simulink library "inp"  (Simulink 7.4)
settings: Solver=ode45  StartTime=0.0  StopTime=10.0  RelTol=1e-3
undefined symbols (not defined in the file): AINP_BrkPedalInterp_X_bar, C_TASK_10MS_S, ENUM_SHIFTER_D, ENUM_SHIFTER_N, ENUM_SHIFTER_P, ENUM_SHIFTER_R, KINP_BonnetCloseVehSpdThre_kph, KINP_EDUCoolantTempFilTm_s, KINP_EDUOilPressureFilTm_s, KINP_EDUOilTempFilTm_s, KINP_EDUSynchDisp_mm, KINP_EDUSynchPosnPWMDC_pct_LowerLimit, KINP_EDUSynchPosnPWMDC_pct_ovrdflg, KINP_EDUSynchPosnPWMDC_pct_ovrdval, KINP_EDUSynchPosnPWMDC_pct_UpperLimit, KINP_ShifterPosConfirmD_s, KINP_ShifterPosConfirmN_s, KINP_ShifterPosConfirmP_s, KINP_ShifterPosConfirmR_s, KINP_SingleAccPedalFltRateLim_pct, KINP_TMSpd2VehSpdSigNeg_rpm, KINP_TMSpd2VehSpdSigPos_rpm, KINP_ValidCheck_EDUSynchPosnPWMDC_dec, KINP_ValidCheck_EDUSynchPosnPWMDC_inc, KINP_ValidCheck_EDUSynchPosnPWMDC_lim, KINP_VehSpdSigKeepThres_kph, KPH2MPS, MIN2SEC, MINP_BrkPedalInterp_pct, MPS2KPH, PI, seat_version_control_block_callbacks, TIRE_RADIUS
libraries: inp_lib x166, hcu_lib x4, simulink x1
(part 4 of 9)

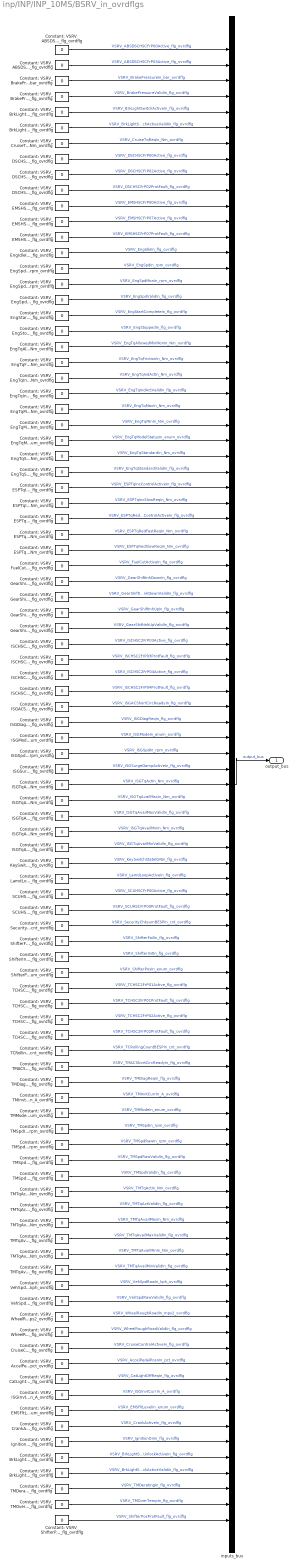
== system inp/INP/INP_10MS/BSRV_in_ovrdflgs ==
  Constant: VSRV_ABSDSCHSCFrP00Active_flg_ovrdflg : Constant  Value=0  OutDataTypeMode=boolean  OutDataTypeStr=boolean
  Constant: VSRV_ABSDSCHSCFrP03Active_flg_ovrdflg : Constant  Value=0  OutDataTypeMode=boolean  OutDataTypeStr=boolean
  Constant: VSRV_AccelPedalPosnIn_pct_ovrdflg : Constant  Value=0  OutDataTypeMode=boolean  OutDataTypeStr=boolean
  Constant: VSRV_BrakePressureIn_bar_ovrdflg : Constant  Value=0  OutDataTypeMode=boolean  OutDataTypeStr=boolean
  Constant: VSRV_BrakePressureValidIn_flg_ovrdflg : Constant  Value=0  OutDataTypeMode=boolean  OutDataTypeStr=boolean
  Constant: VSRV_BrkLightSWPUnlockActiveIn_flg_ovrdflg : Constant  Value=0  OutDataTypeMode=boolean  OutDataTypeStr=boolean
  Constant: VSRV_BrkLightSWPUnlockActiveValidIn_flg_ovrdflg : Constant  Value=0  OutDataTypeMode=boolean  OutDataTypeStr=boolean
  Constant: VSRV_BrkLightSwitchActiveIn_flg_ovrdflg : Constant  Value=0  OutDataTypeMode=boolean  OutDataTypeStr=boolean
  Constant: VSRV_BrkLightSwitchActiveValidIn_flg_ovrdflg : Constant  Value=0  OutDataTypeMode=boolean  OutDataTypeStr=boolean
  Constant: VSRV_CatLightOffReqIn_flg_ovrdflg : Constant  Value=0  OutDataTypeMode=boolean  OutDataTypeStr=boolean
  Constant: VSRV_CrankActiveIn_flg_ovrdflg : Constant  Value=0  OutDataTypeMode=boolean  OutDataTypeStr=boolean
  Constant: VSRV_CruiseControlActiveIn_flg_ovrdflg : Constant  Value=0  OutDataTypeMode=boolean  OutDataTypeStr=boolean
  Constant: VSRV_CruiseTqReqIn_Nm_ovrdflg : Constant  Value=0  OutDataTypeMode=boolean  OutDataTypeStr=boolean
  Constant: VSRV_DSCHSCFrP00Active_flg_ovrdflg : Constant  Value=0  OutDataTypeMode=boolean  OutDataTypeStr=boolean
  Constant: VSRV_DSCHSCFrP02Active_flg_ovrdflg : Constant  Value=0  OutDataTypeMode=boolean  OutDataTypeStr=boolean
  Constant: VSRV_DSCHSCFrP02ProtFault_flg_ovrdflg : Constant  Value=0  OutDataTypeMode=boolean  OutDataTypeStr=boolean
  Constant: VSRV_EMSFltLevelIn_enum_ovrdflg : Constant  Value=0  OutDataTypeMode=boolean  OutDataTypeStr=boolean
  Constant: VSRV_EMSHSCFrP00Active_flg_ovrdflg : Constant  Value=0  OutDataTypeMode=boolean  OutDataTypeStr=boolean
  Constant: VSRV_EMSHSCFrP07Active_flg_ovrdflg : Constant  Value=0  OutDataTypeMode=boolean  OutDataTypeStr=boolean
  Constant: VSRV_EMSHSCFrP07ProtFault_flg_ovrdflg : Constant  Value=0  OutDataTypeMode=boolean  OutDataTypeStr=boolean
  Constant: VSRV_ESPTqIncControlActiveIn_flg_ovrdflg : Constant  Value=0  OutDataTypeMode=boolean  OutDataTypeStr=boolean
  Constant: VSRV_ESPTqIncSlowReqIn_Nm_ovrdflg : Constant  Value=0  OutDataTypeMode=boolean  OutDataTypeStr=boolean
  Constant: VSRV_ESPTqRedControlActiveIn_flg_ovrdflg : Constant  Value=0  OutDataTypeMode=boolean  OutDataTypeStr=boolean
  Constant: VSRV_ESPTqRedFastReqIn_Nm_ovrdflg : Constant  Value=0  OutDataTypeMode=boolean  OutDataTypeStr=boolean
  Constant: VSRV_ESPTqRedSlowReqIn_Nm_ovrdflg : Constant  Value=0  OutDataTypeMode=boolean  OutDataTypeStr=boolean
  Constant: VSRV_EngIdleIn_flg_ovrdflg : Constant  Value=0  OutDataTypeMode=boolean  OutDataTypeStr=boolean
  Constant: VSRV_EngSpdIn_rpm_ovrdflg : Constant  Value=0  OutDataTypeMode=boolean  OutDataTypeStr=boolean
  Constant: VSRV_EngSpdMonIn_rpm_ovrdflg : Constant  Value=0  OutDataTypeMode=boolean  OutDataTypeStr=boolean
  Constant: VSRV_EngSpdValidIn_flg_ovrdflg : Constant  Value=0  OutDataTypeMode=boolean  OutDataTypeStr=boolean
  Constant: VSRV_EngStartCompleteIn_flg_ovrdflg : Constant  Value=0  OutDataTypeMode=boolean  OutDataTypeStr=boolean
  Constant: VSRV_EngStoppedIn_flg_ovrdflg : Constant  Value=0  OutDataTypeMode=boolean  OutDataTypeStr=boolean
  Constant: VSRV_EngTqAllowedMinMonIn_Nm_ovrdflg : Constant  Value=0  OutDataTypeMode=boolean  OutDataTypeStr=boolean
  Constant: VSRV_EngTqFrictionIn_Nm_ovrdflg : Constant  Value=0  OutDataTypeMode=boolean  OutDataTypeStr=boolean
  Constant: VSRV_EngTqIndActIn_Nm_ovrdflg : Constant  Value=0  OutDataTypeMode=boolean  OutDataTypeStr=boolean
  Constant: VSRV_EngTqIndActValidIn_flg_ovrdflg : Constant  Value=0  OutDataTypeMode=boolean  OutDataTypeStr=boolean
  Constant: VSRV_EngTqMaxIn_Nm_ovrdflg : Constant  Value=0  OutDataTypeMode=boolean  OutDataTypeStr=boolean
  Constant: VSRV_EngTqMinIn_Nm_ovrdflg : Constant  Value=0  OutDataTypeMode=boolean  OutDataTypeStr=boolean
  Constant: VSRV_EngTqModelStatusIn_enum_ovrdflg : Constant  Value=0  OutDataTypeMode=boolean  OutDataTypeStr=boolean
  Constant: VSRV_EngTqStandardIn_Nm_ovrdflg : Constant  Value=0  OutDataTypeMode=boolean  OutDataTypeStr=boolean
  Constant: VSRV_EngTqStandardValidIn_flg_ovrdflg : Constant  Value=0  OutDataTypeMode=boolean  OutDataTypeStr=boolean
  Constant: VSRV_FuelCutActiveIn_flg_ovrdflg : Constant  Value=0  OutDataTypeMode=boolean  OutDataTypeStr=boolean
  Constant: VSRV_GearShiftInhDownIn_flg_ovrdflg : Constant  Value=0  OutDataTypeMode=boolean  OutDataTypeStr=boolean
  Constant: VSRV_GearShiftInhDownValidIn_flg_ovrdflg : Constant  Value=0  OutDataTypeMode=boolean  OutDataTypeStr=boolean
  Constant: VSRV_GearShiftInhUpIn_flg_ovrdflg : Constant  Value=0  OutDataTypeMode=boolean  OutDataTypeStr=boolean
  Constant: VSRV_GearShiftInhUpValidIn_flg_ovrdflg : Constant  Value=0  OutDataTypeMode=boolean  OutDataTypeStr=boolean
  Constant: VSRV_ISCHSC2FrP03Active_flg_ovrdflg : Constant  Value=0  OutDataTypeMode=boolean  OutDataTypeStr=boolean
  Constant: VSRV_ISCHSC2FrP03ProtFault_flg_ovrdflg : Constant  Value=0  OutDataTypeMode=boolean  OutDataTypeStr=boolean
  Constant: VSRV_ISCHSC2FrP04Active_flg_ovrdflg : Constant  Value=0  OutDataTypeMode=boolean  OutDataTypeStr=boolean
  Constant: VSRV_ISCHSC2FrP04ProtFault_flg_ovrdflg : Constant  Value=0  OutDataTypeMode=boolean  OutDataTypeStr=boolean
  Constant: VSRV_ISGACShortCircReadyIn_flg_ovrdflg : Constant  Value=0  OutDataTypeMode=boolean  OutDataTypeStr=boolean
  Constant: VSRV_ISGDiagReqIn_flg_ovrdflg : Constant  Value=0  OutDataTypeMode=boolean  OutDataTypeStr=boolean
  Constant: VSRV_ISGInvtCurrIn_A_ovrdflg : Constant  Value=0  OutDataTypeMode=boolean  OutDataTypeStr=boolean
  Constant: VSRV_ISGModeIn_enum_ovrdflg : Constant  Value=0  OutDataTypeMode=boolean  OutDataTypeStr=boolean
  Constant: VSRV_ISGSpdIn_rpm_ovrdflg : Constant  Value=0  OutDataTypeMode=boolean  OutDataTypeStr=boolean
  Constant: VSRV_ISGSurgeDampActiveIn_flg_ovrdflg : Constant  Value=0  OutDataTypeMode=boolean  OutDataTypeStr=boolean
  Constant: VSRV_ISGTqActIn_Nm_ovrdflg : Constant  Value=0  OutDataTypeMode=boolean  OutDataTypeStr=boolean
  Constant: VSRV_ISGTqAvailMaxIn_Nm_ovrdflg : Constant  Value=0  OutDataTypeMode=boolean  OutDataTypeStr=boolean
  Constant: VSRV_ISGTqAvailMaxValidIn_flg_ovrdflg : Constant  Value=0  OutDataTypeMode=boolean  OutDataTypeStr=boolean
  Constant: VSRV_ISGTqAvailMinIn_Nm_ovrdflg : Constant  Value=0  OutDataTypeMode=boolean  OutDataTypeStr=boolean
  Constant: VSRV_ISGTqAvailMinValidIn_flg_ovrdflg : Constant  Value=0  OutDataTypeMode=boolean  OutDataTypeStr=boolean
  Constant: VSRV_IgnitionOnIn_flg_ovrdflg : Constant  Value=0  OutDataTypeMode=boolean  OutDataTypeStr=boolean
  Constant: VSRV_KeySwitchStateIGNIn_flg_ovrdflg : Constant  Value=0  OutDataTypeMode=boolean  OutDataTypeStr=boolean
  Constant: VSRV_LamdLoopActiveIn_flg_ovrdflg : Constant  Value=0  OutDataTypeMode=boolean  OutDataTypeStr=boolean
  Constant: VSRV_SCUHSCFrP00Active_flg_ovrdflg : Constant  Value=0  OutDataTypeMode=boolean  OutDataTypeStr=boolean
  Constant: VSRV_SCUHSCFrP00ProtFault_flg_ovrdflg : Constant  Value=0  OutDataTypeMode=boolean  OutDataTypeStr=boolean
  Constant: VSRV_SecurityChksumBESPIn_cnt_ovrdflg : Constant  Value=0  OutDataTypeMode=boolean  OutDataTypeStr=boolean
  Constant: VSRV_ShifterFailIn_flg_ovrdflg : Constant  Value=0  OutDataTypeMode=boolean  OutDataTypeStr=boolean
  Constant: VSRV_ShifterInitIn_flg_ovrdflg : Constant  Value=0  OutDataTypeMode=boolean  OutDataTypeStr=boolean
  Constant: VSRV_ShifterPosIn_enum_ovrdflg : Constant  Value=0  OutDataTypeMode=boolean  OutDataTypeStr=boolean
  Constant: VSRV_ShifterPosProtFault_flg_ovrdflg : Constant  Value=0  OutDataTypeMode=boolean  OutDataTypeStr=boolean
  Constant: VSRV_TCHSC2FrP01Active_flg_ovrdflg : Constant  Value=0  OutDataTypeMode=boolean  OutDataTypeStr=boolean
  Constant: VSRV_TCHSC2FrP01ProtFault_flg_ovrdflg : Constant  Value=0  OutDataTypeMode=boolean  OutDataTypeStr=boolean
  Constant: VSRV_TCHSC2FrP02Active_flg_ovrdflg : Constant  Value=0  OutDataTypeMode=boolean  OutDataTypeStr=boolean
  Constant: VSRV_TCHSC2FrP02ProtFault_flg_ovrdflg : Constant  Value=0  OutDataTypeMode=boolean  OutDataTypeStr=boolean
  Constant: VSRV_TCRollingCountBESPIn_cnt_ovrdflg : Constant  Value=0  OutDataTypeMode=boolean  OutDataTypeStr=boolean
  Constant: VSRV_TMACShortCircReadyIn_flg_ovrdflg : Constant  Value=0  OutDataTypeMode=boolean  OutDataTypeStr=boolean
  Constant: VSRV_TMDeratingIn_flg_ovrdflg : Constant  Value=0  OutDataTypeMode=boolean  OutDataTypeStr=boolean
  Constant: VSRV_TMDiagReqIn_flg_ovrdflg : Constant  Value=0  OutDataTypeMode=boolean  OutDataTypeStr=boolean
  Constant: VSRV_TMInvtCurrIn_A_ovrdflg : Constant  Value=0  OutDataTypeMode=boolean  OutDataTypeStr=boolean
  Constant: VSRV_TMModeIn_enum_ovrdflg : Constant  Value=0  OutDataTypeMode=boolean  OutDataTypeStr=boolean
  Constant: VSRV_TMOverTempIn_flg_ovrdflg : Constant  Value=0  OutDataTypeMode=boolean  OutDataTypeStr=boolean
  Constant: VSRV_TMSpdIn_rpm_ovrdflg : Constant  Value=0  OutDataTypeMode=boolean  OutDataTypeStr=boolean
  Constant: VSRV_TMSpdRawIn_rpm_ovrdflg : Constant  Value=0  OutDataTypeMode=boolean  OutDataTypeStr=boolean
  Constant: VSRV_TMSpdRawValidIn_flg_ovrdflg : Constant  Value=0  OutDataTypeMode=boolean  OutDataTypeStr=boolean
  Constant: VSRV_TMSpdValidIn_flg_ovrdflg : Constant  Value=0  OutDataTypeMode=boolean  OutDataTypeStr=boolean
  Constant: VSRV_TMTqActIn_Nm_ovrdflg : Constant  Value=0  OutDataTypeMode=boolean  OutDataTypeStr=boolean
  Constant: VSRV_TMTqActValidIn_flg_ovrdflg : Constant  Value=0  OutDataTypeMode=boolean  OutDataTypeStr=boolean
  Constant: VSRV_TMTqAvailMaxIn_Nm_ovrdflg : Constant  Value=0  OutDataTypeMode=boolean  OutDataTypeStr=boolean
  Constant: VSRV_TMTqAvailMaxValidIn_flg_ovrdflg : Constant  Value=0  OutDataTypeMode=boolean  OutDataTypeStr=boolean
  Constant: VSRV_TMTqAvailMinIn_Nm_ovrdflg : Constant  Value=0  OutDataTypeMode=boolean  OutDataTypeStr=boolean
  Constant: VSRV_TMTqAvailMinValidIn_flg_ovrdflg : Constant  Value=0  OutDataTypeMode=boolean  OutDataTypeStr=boolean
  Constant: VSRV_VehSpdRawIn_kph_ovrdflg : Constant  Value=0  OutDataTypeMode=boolean  OutDataTypeStr=boolean
  Constant: VSRV_VehSpdRawValidIn_flg_ovrdflg : Constant  Value=0  OutDataTypeMode=boolean  OutDataTypeStr=boolean
  Constant: VSRV_WheelRoughRoadIn_mps2_ovrdflg : Constant  Value=0  OutDataTypeMode=boolean  OutDataTypeStr=boolean
  Constant: VSRV_WheelRoughRoadValidIn_flg_ovrdflg : Constant  Value=0  OutDataTypeMode=boolean  OutDataTypeStr=boolean
  inputs_bus : BusCreator  Inputs=95
  output_bus : Outport
  wires:
  Constant: VSRV_ShifterPosProtFault_flg_ovrdflg/1 -> inputs_bus/95  "VSRV_ShifterPosProtFault_flg_ovrdflg"
  Constant: VSRV_TMOverTempIn_flg_ovrdflg/1 -> inputs_bus/94  "VSRV_TMOverTempIn_flg_ovrdflg"
  Constant: VSRV_TMDeratingIn_flg_ovrdflg/1 -> inputs_bus/93  "VSRV_TMDeratingIn_flg_ovrdflg"
  Constant: VSRV_BrkLightSWPUnlockActiveValidIn_flg_ovrdflg/1 -> inputs_bus/92  "VSRV_BrkLightSWPUnlockActiveValidIn_flg_ovrdflg"
  Constant: VSRV_BrkLightSWPUnlockActiveIn_flg_ovrdflg/1 -> inputs_bus/91  "VSRV_BrkLightSWPUnlockActiveIn_flg_ovrdflg"
  Constant: VSRV_IgnitionOnIn_flg_ovrdflg/1 -> inputs_bus/90  "VSRV_IgnitionOnIn_flg_ovrdflg"
  Constant: VSRV_CrankActiveIn_flg_ovrdflg/1 -> inputs_bus/89  "VSRV_CrankActiveIn_flg_ovrdflg"
  Constant: VSRV_WheelRoughRoadValidIn_flg_ovrdflg/1 -> inputs_bus/83  "VSRV_WheelRoughRoadValidIn_flg_ovrdflg"
  Constant: VSRV_WheelRoughRoadIn_mps2_ovrdflg/1 -> inputs_bus/82  "VSRV_WheelRoughRoadIn_mps2_ovrdflg"
  Constant: VSRV_VehSpdRawValidIn_flg_ovrdflg/1 -> inputs_bus/81  "VSRV_VehSpdRawValidIn_flg_ovrdflg"
  Constant: VSRV_VehSpdRawIn_kph_ovrdflg/1 -> inputs_bus/80  "VSRV_VehSpdRawIn_kph_ovrdflg"
  Constant: VSRV_TMTqAvailMinValidIn_flg_ovrdflg/1 -> inputs_bus/79  "VSRV_TMTqAvailMinValidIn_flg_ovrdflg"
  Constant: VSRV_TMTqAvailMinIn_Nm_ovrdflg/1 -> inputs_bus/78  "VSRV_TMTqAvailMinIn_Nm_ovrdflg"
  Constant: VSRV_TMTqAvailMaxValidIn_flg_ovrdflg/1 -> inputs_bus/77  "VSRV_TMTqAvailMaxValidIn_flg_ovrdflg"
  Constant: VSRV_TMTqAvailMaxIn_Nm_ovrdflg/1 -> inputs_bus/76  "VSRV_TMTqAvailMaxIn_Nm_ovrdflg"
  Constant: VSRV_TMTqActValidIn_flg_ovrdflg/1 -> inputs_bus/75  "VSRV_TMTqActValidIn_flg_ovrdflg"
  Constant: VSRV_TMTqActIn_Nm_ovrdflg/1 -> inputs_bus/74  "VSRV_TMTqActIn_Nm_ovrdflg"
  Constant: VSRV_TMSpdValidIn_flg_ovrdflg/1 -> inputs_bus/73  "VSRV_TMSpdValidIn_flg_ovrdflg"
  Constant: VSRV_TMSpdRawValidIn_flg_ovrdflg/1 -> inputs_bus/72  "VSRV_TMSpdRawValidIn_flg_ovrdflg"
  Constant: VSRV_TMSpdRawIn_rpm_ovrdflg/1 -> inputs_bus/71  "VSRV_TMSpdRawIn_rpm_ovrdflg"
  Constant: VSRV_TMSpdIn_rpm_ovrdflg/1 -> inputs_bus/70  "VSRV_TMSpdIn_rpm_ovrdflg"
  Constant: VSRV_TMModeIn_enum_ovrdflg/1 -> inputs_bus/69  "VSRV_TMModeIn_enum_ovrdflg"
  Constant: VSRV_TMInvtCurrIn_A_ovrdflg/1 -> inputs_bus/68  "VSRV_TMInvtCurrIn_A_ovrdflg"
  Constant: VSRV_TMDiagReqIn_flg_ovrdflg/1 -> inputs_bus/67  "VSRV_TMDiagReqIn_flg_ovrdflg"
  Constant: VSRV_TMACShortCircReadyIn_flg_ovrdflg/1 -> inputs_bus/66  "VSRV_TMACShortCircReadyIn_flg_ovrdflg"
  Constant: VSRV_TCRollingCountBESPIn_cnt_ovrdflg/1 -> inputs_bus/65  "VSRV_TCRollingCountBESPIn_cnt_ovrdflg"
  Constant: VSRV_TCHSC2FrP02ProtFault_flg_ovrdflg/1 -> inputs_bus/64  "VSRV_TCHSC2FrP02ProtFault_flg_ovrdflg"
  Constant: VSRV_TCHSC2FrP02Active_flg_ovrdflg/1 -> inputs_bus/63  "VSRV_TCHSC2FrP02Active_flg_ovrdflg"
  Constant: VSRV_TCHSC2FrP01ProtFault_flg_ovrdflg/1 -> inputs_bus/62  "VSRV_TCHSC2FrP01ProtFault_flg_ovrdflg"
  Constant: VSRV_TCHSC2FrP01Active_flg_ovrdflg/1 -> inputs_bus/61  "VSRV_TCHSC2FrP01Active_flg_ovrdflg"
  Constant: VSRV_ShifterPosIn_enum_ovrdflg/1 -> inputs_bus/60  "VSRV_ShifterPosIn_enum_ovrdflg"
  Constant: VSRV_ShifterInitIn_flg_ovrdflg/1 -> inputs_bus/59  "VSRV_ShifterInitIn_flg_ovrdflg"
  Constant: VSRV_ShifterFailIn_flg_ovrdflg/1 -> inputs_bus/58  "VSRV_ShifterFailIn_flg_ovrdflg"
  Constant: VSRV_SecurityChksumBESPIn_cnt_ovrdflg/1 -> inputs_bus/57  "VSRV_SecurityChksumBESPIn_cnt_ovrdflg"
  Constant: VSRV_SCUHSCFrP00ProtFault_flg_ovrdflg/1 -> inputs_bus/56  "VSRV_SCUHSCFrP00ProtFault_flg_ovrdflg"
  Constant: VSRV_SCUHSCFrP00Active_flg_ovrdflg/1 -> inputs_bus/55  "VSRV_SCUHSCFrP00Active_flg_ovrdflg"
  Constant: VSRV_LamdLoopActiveIn_flg_ovrdflg/1 -> inputs_bus/54  "VSRV_LamdLoopActiveIn_flg_ovrdflg"
  Constant: VSRV_KeySwitchStateIGNIn_flg_ovrdflg/1 -> inputs_bus/53  "VSRV_KeySwitchStateIGNIn_flg_ovrdflg"
  Constant: VSRV_ISGTqAvailMinValidIn_flg_ovrdflg/1 -> inputs_bus/52  "VSRV_ISGTqAvailMinValidIn_flg_ovrdflg"
  Constant: VSRV_ISGTqAvailMinIn_Nm_ovrdflg/1 -> inputs_bus/51  "VSRV_ISGTqAvailMinIn_Nm_ovrdflg"
  Constant: VSRV_ISGTqAvailMaxValidIn_flg_ovrdflg/1 -> inputs_bus/50  "VSRV_ISGTqAvailMaxValidIn_flg_ovrdflg"
  Constant: VSRV_ISGTqAvailMaxIn_Nm_ovrdflg/1 -> inputs_bus/49  "VSRV_ISGTqAvailMaxIn_Nm_ovrdflg"
  Constant: VSRV_ISGTqActIn_Nm_ovrdflg/1 -> inputs_bus/48  "VSRV_ISGTqActIn_Nm_ovrdflg"
  Constant: VSRV_ISGSurgeDampActiveIn_flg_ovrdflg/1 -> inputs_bus/47  "VSRV_ISGSurgeDampActiveIn_flg_ovrdflg"
  Constant: VSRV_ISGSpdIn_rpm_ovrdflg/1 -> inputs_bus/46  "VSRV_ISGSpdIn_rpm_ovrdflg"
  Constant: VSRV_ISGModeIn_enum_ovrdflg/1 -> inputs_bus/45  "VSRV_ISGModeIn_enum_ovrdflg"
  Constant: VSRV_ISGDiagReqIn_flg_ovrdflg/1 -> inputs_bus/44  "VSRV_ISGDiagReqIn_flg_ovrdflg"
  Constant: VSRV_ISGACShortCircReadyIn_flg_ovrdflg/1 -> inputs_bus/43  "VSRV_ISGACShortCircReadyIn_flg_ovrdflg"
  Constant: VSRV_ISCHSC2FrP04ProtFault_flg_ovrdflg/1 -> inputs_bus/42  "VSRV_ISCHSC2FrP04ProtFault_flg_ovrdflg"
  Constant: VSRV_ISCHSC2FrP04Active_flg_ovrdflg/1 -> inputs_bus/41  "VSRV_ISCHSC2FrP04Active_flg_ovrdflg"
  Constant: VSRV_ISCHSC2FrP03ProtFault_flg_ovrdflg/1 -> inputs_bus/40  "VSRV_ISCHSC2FrP03ProtFault_flg_ovrdflg"
  Constant: VSRV_ISCHSC2FrP03Active_flg_ovrdflg/1 -> inputs_bus/39  "VSRV_ISCHSC2FrP03Active_flg_ovrdflg"
  Constant: VSRV_GearShiftInhUpValidIn_flg_ovrdflg/1 -> inputs_bus/38  "VSRV_GearShiftInhUpValidIn_flg_ovrdflg"
  Constant: VSRV_GearShiftInhUpIn_flg_ovrdflg/1 -> inputs_bus/37  "VSRV_GearShiftInhUpIn_flg_ovrdflg"
  Constant: VSRV_GearShiftInhDownValidIn_flg_ovrdflg/1 -> inputs_bus/36  "VSRV_GearShiftInhDownValidIn_flg_ovrdflg"
  Constant: VSRV_GearShiftInhDownIn_flg_ovrdflg/1 -> inputs_bus/35  "VSRV_GearShiftInhDownIn_flg_ovrdflg"
  Constant: VSRV_FuelCutActiveIn_flg_ovrdflg/1 -> inputs_bus/34  "VSRV_FuelCutActiveIn_flg_ovrdflg"
  Constant: VSRV_ESPTqRedSlowReqIn_Nm_ovrdflg/1 -> inputs_bus/33  "VSRV_ESPTqRedSlowReqIn_Nm_ovrdflg"
  Constant: VSRV_ESPTqRedFastReqIn_Nm_ovrdflg/1 -> inputs_bus/32  "VSRV_ESPTqRedFastReqIn_Nm_ovrdflg"
  Constant: VSRV_ESPTqRedControlActiveIn_flg_ovrdflg/1 -> inputs_bus/31  "VSRV_ESPTqRedControlActiveIn_flg_ovrdflg"
  Constant: VSRV_ESPTqIncSlowReqIn_Nm_ovrdflg/1 -> inputs_bus/30  "VSRV_ESPTqIncSlowReqIn_Nm_ovrdflg"
  Constant: VSRV_ESPTqIncControlActiveIn_flg_ovrdflg/1 -> inputs_bus/29  "VSRV_ESPTqIncControlActiveIn_flg_ovrdflg"
  Constant: VSRV_EngTqStandardValidIn_flg_ovrdflg/1 -> inputs_bus/28  "VSRV_EngTqStandardValidIn_flg_ovrdflg"
  Constant: VSRV_EngTqStandardIn_Nm_ovrdflg/1 -> inputs_bus/27  "VSRV_EngTqStandardIn_Nm_ovrdflg"
  Constant: VSRV_EngTqModelStatusIn_enum_ovrdflg/1 -> inputs_bus/26  "VSRV_EngTqModelStatusIn_enum_ovrdflg"
  Constant: VSRV_EngTqMinIn_Nm_ovrdflg/1 -> inputs_bus/25  "VSRV_EngTqMinIn_Nm_ovrdflg"
  Constant: VSRV_EngTqMaxIn_Nm_ovrdflg/1 -> inputs_bus/24  "VSRV_EngTqMaxIn_Nm_ovrdflg"
  Constant: VSRV_EngTqIndActValidIn_flg_ovrdflg/1 -> inputs_bus/23  "VSRV_EngTqIndActValidIn_flg_ovrdflg"
  Constant: VSRV_EngTqIndActIn_Nm_ovrdflg/1 -> inputs_bus/22  "VSRV_EngTqIndActIn_Nm_ovrdflg"
  Constant: VSRV_EngTqFrictionIn_Nm_ovrdflg/1 -> inputs_bus/21  "VSRV_EngTqFrictionIn_Nm_ovrdflg"
  Constant: VSRV_EngTqAllowedMinMonIn_Nm_ovrdflg/1 -> inputs_bus/20  "VSRV_EngTqAllowedMinMonIn_Nm_ovrdflg"
  Constant: VSRV_EngStoppedIn_flg_ovrdflg/1 -> inputs_bus/19  "VSRV_EngStoppedIn_flg_ovrdflg"
  Constant: VSRV_EngStartCompleteIn_flg_ovrdflg/1 -> inputs_bus/18  "VSRV_EngStartCompleteIn_flg_ovrdflg"
  Constant: VSRV_EngSpdValidIn_flg_ovrdflg/1 -> inputs_bus/17  "VSRV_EngSpdValidIn_flg_ovrdflg"
  Constant: VSRV_EngSpdMonIn_rpm_ovrdflg/1 -> inputs_bus/16  "VSRV_EngSpdMonIn_rpm_ovrdflg"
  Constant: VSRV_EngSpdIn_rpm_ovrdflg/1 -> inputs_bus/15  "VSRV_EngSpdIn_rpm_ovrdflg"
  Constant: VSRV_EngIdleIn_flg_ovrdflg/1 -> inputs_bus/14  "VSRV_EngIdleIn_flg_ovrdflg"
  Constant: VSRV_EMSHSCFrP07ProtFault_flg_ovrdflg/1 -> inputs_bus/13  "VSRV_EMSHSCFrP07ProtFault_flg_ovrdflg"
  Constant: VSRV_EMSHSCFrP07Active_flg_ovrdflg/1 -> inputs_bus/12  "VSRV_EMSHSCFrP07Active_flg_ovrdflg"
  Constant: VSRV_EMSHSCFrP00Active_flg_ovrdflg/1 -> inputs_bus/11  "VSRV_EMSHSCFrP00Active_flg_ovrdflg"
  Constant: VSRV_DSCHSCFrP02ProtFault_flg_ovrdflg/1 -> inputs_bus/10  "VSRV_DSCHSCFrP02ProtFault_flg_ovrdflg"
  Constant: VSRV_DSCHSCFrP02Active_flg_ovrdflg/1 -> inputs_bus/9  "VSRV_DSCHSCFrP02Active_flg_ovrdflg"
  Constant: VSRV_DSCHSCFrP00Active_flg_ovrdflg/1 -> inputs_bus/8  "VSRV_DSCHSCFrP00Active_flg_ovrdflg"
  Constant: VSRV_CruiseTqReqIn_Nm_ovrdflg/1 -> inputs_bus/7  "VSRV_CruiseTqReqIn_Nm_ovrdflg"
  Constant: VSRV_BrkLightSwitchActiveValidIn_flg_ovrdflg/1 -> inputs_bus/6  "VSRV_BrkLightSwitchActiveValidIn_flg_ovrdflg"
  Constant: VSRV_BrkLightSwitchActiveIn_flg_ovrdflg/1 -> inputs_bus/5  "VSRV_BrkLightSwitchActiveIn_flg_ovrdflg"
  Constant: VSRV_BrakePressureValidIn_flg_ovrdflg/1 -> inputs_bus/4  "VSRV_BrakePressureValidIn_flg_ovrdflg"
  Constant: VSRV_BrakePressureIn_bar_ovrdflg/1 -> inputs_bus/3  "VSRV_BrakePressureIn_bar_ovrdflg"
  Constant: VSRV_ABSDSCHSCFrP03Active_flg_ovrdflg/1 -> inputs_bus/2  "VSRV_ABSDSCHSCFrP03Active_flg_ovrdflg"
  Constant: VSRV_ABSDSCHSCFrP00Active_flg_ovrdflg/1 -> inputs_bus/1  "VSRV_ABSDSCHSCFrP00Active_flg_ovrdflg"
  inputs_bus/1 -> output_bus/1  "output_bus"
  Constant: VSRV_CruiseControlActiveIn_flg_ovrdflg/1 -> inputs_bus/84  "VSRV_CruiseControlActiveIn_flg_ovrdflg"
  Constant: VSRV_AccelPedalPosnIn_pct_ovrdflg/1 -> inputs_bus/85  "VSRV_AccelPedalPosnIn_pct_ovrdflg"
  Constant: VSRV_CatLightOffReqIn_flg_ovrdflg/1 -> inputs_bus/86  "VSRV_CatLightOffReqIn_flg_ovrdflg"
  Constant: VSRV_ISGInvtCurrIn_A_ovrdflg/1 -> inputs_bus/87  "VSRV_ISGInvtCurrIn_A_ovrdflg"
  Constant: VSRV_EMSFltLevelIn_enum_ovrdflg/1 -> inputs_bus/88  "VSRV_EMSFltLevelIn_enum_ovrdflg"

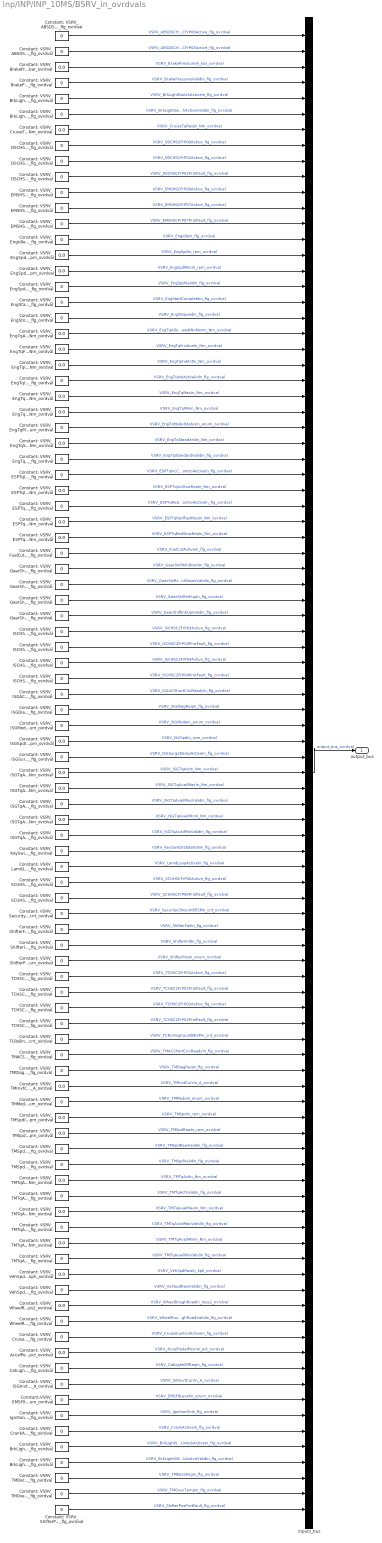
== system inp/INP/INP_10MS/BSRV_in_ovrdvals ==
  Constant: VSRV_ABSDSCHSCFrP00Active_flg_ovrdval : Constant  Value=0  OutDataTypeMode=boolean  OutDataTypeStr=boolean
  Constant: VSRV_ABSDSCHSCFrP03Active_flg_ovrdval : Constant  Value=0  OutDataTypeMode=boolean  OutDataTypeStr=boolean
  Constant: VSRV_AccelPedalPosnMonIn_pct_ovrdval : Constant  Value=0.0  OutDataTypeMode=single  OutDataTypeStr=single
  Constant: VSRV_BrakePressureIn_bar_ovrdval : Constant  Value=0.0  OutDataTypeMode=single  OutDataTypeStr=single
  Constant: VSRV_BrakePressureValidIn_flg_ovrdval : Constant  Value=0  OutDataTypeMode=boolean  OutDataTypeStr=boolean
  Constant: VSRV_BrkLightSWPUnlockActiveIn_flg_ovrdval : Constant  Value=0  OutDataTypeMode=boolean  OutDataTypeStr=boolean
  Constant: VSRV_BrkLightSWPUnlockActiveValidIn_flg_ovrdval : Constant  Value=0  OutDataTypeMode=boolean  OutDataTypeStr=boolean
  Constant: VSRV_BrkLightSwitchActiveIn_flg_ovrdval : Constant  Value=0  OutDataTypeMode=boolean  OutDataTypeStr=boolean
  Constant: VSRV_BrkLightSwitchActiveValidIn_flg_ovrdval : Constant  Value=0  OutDataTypeMode=boolean  OutDataTypeStr=boolean
  Constant: VSRV_CatLightOffReqIn_flg_ovrdval : Constant  Value=0  OutDataTypeMode=boolean  OutDataTypeStr=boolean
  Constant: VSRV_CrankActiveIn_flg_ovrdval : Constant  Value=0  OutDataTypeMode=boolean  OutDataTypeStr=boolean
  Constant: VSRV_CruiseControlActiveIn_flg_ovrdval : Constant  Value=0  OutDataTypeMode=boolean  OutDataTypeStr=boolean
  Constant: VSRV_CruiseTqReqIn_Nm_ovrdval : Constant  Value=0.0  OutDataTypeMode=single  OutDataTypeStr=single
  Constant: VSRV_DSCHSCFrP00Active_flg_ovrdval : Constant  Value=0  OutDataTypeMode=boolean  OutDataTypeStr=boolean
  Constant: VSRV_DSCHSCFrP02Active_flg_ovrdval : Constant  Value=0  OutDataTypeMode=boolean  OutDataTypeStr=boolean
  Constant: VSRV_DSCHSCFrP02ProtFault_flg_ovrdval : Constant  Value=0  OutDataTypeMode=boolean  OutDataTypeStr=boolean
  Constant: VSRV_EMSHSCFrP00Active_flg_ovrdval : Constant  Value=0  OutDataTypeMode=boolean  OutDataTypeStr=boolean
  Constant: VSRV_EMSHSCFrP07Active_flg_ovrdval : Constant  Value=0  OutDataTypeMode=boolean  OutDataTypeStr=boolean
  Constant: VSRV_EMSHSCFrP07ProtFault_flg_ovrdval : Constant  Value=0  OutDataTypeMode=boolean  OutDataTypeStr=boolean
  Constant: VSRV_ESPTqIncControlActiveIn_flg_ovrdval : Constant  Value=0  OutDataTypeMode=boolean  OutDataTypeStr=boolean
  Constant: VSRV_ESPTqIncSlowReqIn_Nm_ovrdval : Constant  Value=0.0  OutDataTypeMode=single  OutDataTypeStr=single
  Constant: VSRV_ESPTqRedControlActiveIn_flg_ovrdval : Constant  Value=0  OutDataTypeMode=boolean  OutDataTypeStr=boolean
  Constant: VSRV_ESPTqRedFastReqIn_Nm_ovrdval : Constant  Value=0.0  OutDataTypeMode=single  OutDataTypeStr=single
  Constant: VSRV_ESPTqRedSlowReqIn_Nm_ovrdval : Constant  Value=0.0  OutDataTypeMode=single  OutDataTypeStr=single
  Constant: VSRV_EngIdleIn_flg_ovrdval : Constant  Value=0  OutDataTypeMode=boolean  OutDataTypeStr=boolean
  Constant: VSRV_EngSpdIn_rpm_ovrdval : Constant  Value=0.0  OutDataTypeMode=single  OutDataTypeStr=single
  Constant: VSRV_EngSpdMonIn_rpm_ovrdval : Constant  Value=0.0  OutDataTypeMode=single  OutDataTypeStr=single
  Constant: VSRV_EngSpdValidIn_flg_ovrdval : Constant  Value=0  OutDataTypeMode=boolean  OutDataTypeStr=boolean
  Constant: VSRV_EngStartCompleteIn_flg_ovrdval : Constant  Value=0  OutDataTypeMode=boolean  OutDataTypeStr=boolean
  Constant: VSRV_EngStoppedIn_flg_ovrdval : Constant  Value=0  OutDataTypeMode=boolean  OutDataTypeStr=boolean
  Constant: VSRV_EngTqAllowedMinMonIn_Nm_ovrdval : Constant  Value=0.0  OutDataTypeMode=single  OutDataTypeStr=single
  Constant: VSRV_EngTqFrictionIn_Nm_ovrdval : Constant  Value=0.0  OutDataTypeMode=single  OutDataTypeStr=single
  Constant: VSRV_EngTqIndActIn_Nm_ovrdval : Constant  Value=0.0  OutDataTypeMode=single  OutDataTypeStr=single
  Constant: VSRV_EngTqIndActValidIn_flg_ovrdval : Constant  Value=0  OutDataTypeMode=boolean  OutDataTypeStr=boolean
  Constant: VSRV_EngTqMaxIn_Nm_ovrdval : Constant  Value=0.0  OutDataTypeMode=single  OutDataTypeStr=single
  Constant: VSRV_EngTqMinIn_Nm_ovrdval : Constant  Value=0.0  OutDataTypeMode=single  OutDataTypeStr=single
  Constant: VSRV_EngTqModelStatusIn_enum_ovrdval : Constant  Value=0  OutDataTypeMode=uint8  OutDataTypeStr=uint8
  Constant: VSRV_EngTqStandardIn_Nm_ovrdval : Constant  Value=0.0  OutDataTypeMode=single  OutDataTypeStr=single
  Constant: VSRV_EngTqStandardValidIn_flg_ovrdval : Constant  Value=0  OutDataTypeMode=boolean  OutDataTypeStr=boolean
  Constant: VSRV_FuelCutActiveIn_flg_ovrdval : Constant  Value=0  OutDataTypeMode=boolean  OutDataTypeStr=boolean
  Constant: VSRV_GearShiftInhDownIn_flg_ovrdval : Constant  Value=0  OutDataTypeMode=boolean  OutDataTypeStr=boolean
  Constant: VSRV_GearShiftInhDownValidIn_flg_ovrdval : Constant  Value=0  OutDataTypeMode=boolean  OutDataTypeStr=boolean
  Constant: VSRV_GearShiftInhUpIn_flg_ovrdval : Constant  Value=0  OutDataTypeMode=boolean  OutDataTypeStr=boolean
  Constant: VSRV_GearShiftInhUpValidIn_flg_ovrdval : Constant  Value=0  OutDataTypeMode=boolean  OutDataTypeStr=boolean
  Constant: VSRV_ISCHSC2FrP03Active_flg_ovrdval : Constant  Value=0  OutDataTypeMode=boolean  OutDataTypeStr=boolean
  Constant: VSRV_ISCHSC2FrP03ProtFault_flg_ovrdval : Constant  Value=0  OutDataTypeMode=boolean  OutDataTypeStr=boolean
  Constant: VSRV_ISCHSC2FrP04Active_flg_ovrdval : Constant  Value=0  OutDataTypeMode=boolean  OutDataTypeStr=boolean
  Constant: VSRV_ISCHSC2FrP04ProtFault_flg_ovrdval : Constant  Value=0  OutDataTypeMode=boolean  OutDataTypeStr=boolean
  Constant: VSRV_ISGACShortCircReadyIn_flg_ovrdval : Constant  Value=0  OutDataTypeMode=boolean  OutDataTypeStr=boolean
  Constant: VSRV_ISGDiagReqIn_flg_ovrdval : Constant  Value=0  OutDataTypeMode=boolean  OutDataTypeStr=boolean
  Constant: VSRV_ISGInvtCurrIn_A_ovrdval : Constant  Value=0  OutDataTypeMode=single  OutDataTypeStr=single
  Constant: VSRV_ISGModeIn_enum_ovrdval : Constant  Value=0  OutDataTypeMode=uint8  OutDataTypeStr=uint8
  Constant: VSRV_ISGSpdIn_rpm_ovrdval : Constant  Value=0.0  OutDataTypeMode=single  OutDataTypeStr=single
  Constant: VSRV_ISGSurgeDampActiveIn_flg_ovrdval : Constant  Value=0  OutDataTypeMode=boolean  OutDataTypeStr=boolean
  Constant: VSRV_ISGTqActIn_Nm_ovrdval : Constant  Value=0.0  OutDataTypeMode=single  OutDataTypeStr=single
  Constant: VSRV_ISGTqAvailMaxIn_Nm_ovrdval : Constant  Value=0.0  OutDataTypeMode=single  OutDataTypeStr=single
  Constant: VSRV_ISGTqAvailMaxValidIn_flg_ovrdval : Constant  Value=0  OutDataTypeMode=boolean  OutDataTypeStr=boolean
  Constant: VSRV_ISGTqAvailMinIn_Nm_ovrdval : Constant  Value=0.0  OutDataTypeMode=single  OutDataTypeStr=single
  Constant: VSRV_ISGTqAvailMinValidIn_flg_ovrdval : Constant  Value=0  OutDataTypeMode=boolean  OutDataTypeStr=boolean
  Constant: VSRV_IgnitionOnIn_flg_ovrdval : Constant  Value=0  OutDataTypeMode=boolean  OutDataTypeStr=boolean
  Constant: VSRV_KeySwitchStateIGNIn_flg_ovrdval : Constant  Value=0  OutDataTypeMode=boolean  OutDataTypeStr=boolean
  Constant: VSRV_LamdLoopActiveIn_flg_ovrdval : Constant  Value=0  OutDataTypeMode=boolean  OutDataTypeStr=boolean
  Constant: VSRV_SCUHSCFrP00Active_flg_ovrdval : Constant  Value=0  OutDataTypeMode=boolean  OutDataTypeStr=boolean
  Constant: VSRV_SCUHSCFrP00ProtFault_flg_ovrdval : Constant  Value=0  OutDataTypeMode=boolean  OutDataTypeStr=boolean
  Constant: VSRV_SecurityChksumBESPIn_cnt_ovrdval : Constant  Value=0  OutDataTypeMode=uint8  OutDataTypeStr=uint8
  Constant: VSRV_ShifterFailIn_flg_ovrdval : Constant  Value=0  OutDataTypeMode=boolean  OutDataTypeStr=boolean
  Constant: VSRV_ShifterInitIn_flg_ovrdval : Constant  Value=0  OutDataTypeMode=boolean  OutDataTypeStr=boolean
  Constant: VSRV_ShifterPosIn_enum_ovrdval : Constant  Value=0  OutDataTypeMode=uint8  OutDataTypeStr=uint8
  Constant: VSRV_ShifterPosProtFault_flg_ovrdval : Constant  Value=0  OutDataTypeMode=boolean  OutDataTypeStr=boolean
  Constant: VSRV_TCHSC2FrP01Active_flg_ovrdval : Constant  Value=0  OutDataTypeMode=boolean  OutDataTypeStr=boolean
  Constant: VSRV_TCHSC2FrP01ProtFault_flg_ovrdval : Constant  Value=0  OutDataTypeMode=boolean  OutDataTypeStr=boolean
  Constant: VSRV_TCHSC2FrP02Active_flg_ovrdval : Constant  Value=0  OutDataTypeMode=boolean  OutDataTypeStr=boolean
  Constant: VSRV_TCHSC2FrP02ProtFault_flg_ovrdval : Constant  Value=0  OutDataTypeMode=boolean  OutDataTypeStr=boolean
  Constant: VSRV_TCRollingCountBESPIn_cnt_ovrdval : Constant  Value=0  OutDataTypeMode=uint8  OutDataTypeStr=uint8
  Constant: VSRV_TMACShortCircReadyIn_flg_ovrdval : Constant  Value=0  OutDataTypeMode=boolean  OutDataTypeStr=boolean
  Constant: VSRV_TMDeratingIn_flg_ovrdval : Constant  Value=0  OutDataTypeMode=boolean  OutDataTypeStr=boolean
  Constant: VSRV_TMDiagReqIn_flg_ovrdval : Constant  Value=0  OutDataTypeMode=boolean  OutDataTypeStr=boolean
  Constant: VSRV_TMInvtCurrIn_A_ovrdval : Constant  Value=0.0  OutDataTypeMode=single  OutDataTypeStr=single
  Constant: VSRV_TMModeIn_enum_ovrdval : Constant  Value=0  OutDataTypeMode=uint8  OutDataTypeStr=uint8
  Constant: VSRV_TMOverTempIn_flg_ovrdval : Constant  Value=0  OutDataTypeMode=boolean  OutDataTypeStr=boolean
  Constant: VSRV_TMSpdIn_rpm_ovrdval : Constant  Value=0.0  OutDataTypeMode=single  OutDataTypeStr=single
  Constant: VSRV_TMSpdRawIn_rpm_ovrdval : Constant  Value=0.0  OutDataTypeMode=single  OutDataTypeStr=single
  Constant: VSRV_TMSpdRawValidIn_flg_ovrdval : Constant  Value=0  OutDataTypeMode=boolean  OutDataTypeStr=boolean
  Constant: VSRV_TMSpdValidIn_flg_ovrdval : Constant  Value=0  OutDataTypeMode=boolean  OutDataTypeStr=boolean
  Constant: VSRV_TMTqActIn_Nm_ovrdval : Constant  Value=0.0  OutDataTypeMode=single  OutDataTypeStr=single
  Constant: VSRV_TMTqActValidIn_flg_ovrdval : Constant  Value=0  OutDataTypeMode=boolean  OutDataTypeStr=boolean
  Constant: VSRV_TMTqAvailMaxIn_Nm_ovrdval : Constant  Value=0.0  OutDataTypeMode=single  OutDataTypeStr=single
  Constant: VSRV_TMTqAvailMaxValidIn_flg_ovrdval : Constant  Value=0  OutDataTypeMode=boolean  OutDataTypeStr=boolean
  Constant: VSRV_TMTqAvailMinIn_Nm_ovrdval : Constant  Value=0.0  OutDataTypeMode=single  OutDataTypeStr=single
  Constant: VSRV_TMTqAvailMinValidIn_flg_ovrdval : Constant  Value=0  OutDataTypeMode=boolean  OutDataTypeStr=boolean
  Constant: VSRV_VehSpdRawIn_kph_ovrdval : Constant  Value=0.0  OutDataTypeMode=single  OutDataTypeStr=single
  Constant: VSRV_VehSpdRawValidIn_flg_ovrdval : Constant  Value=0  OutDataTypeMode=boolean  OutDataTypeStr=boolean
  Constant: VSRV_WheelRoughRoadIn_mps2_ovrdval : Constant  Value=0.0  OutDataTypeMode=single  OutDataTypeStr=single
  Constant: VSRV_WheelRoughRoadValidIn_flg_ovrdval : Constant  Value=0  OutDataTypeMode=boolean  OutDataTypeStr=boolean
  Constant:VSRV_EMSFltLevelIn_enum_ovrdval : Constant  Value=0  OutDataTypeMode=uint8  OutDataTypeStr=uint8
  inputs_bus : BusCreator  Inputs=95
  output_bus : Outport
  wires:
  Constant: VSRV_ShifterPosProtFault_flg_ovrdval/1 -> inputs_bus/95  "VSRV_ShifterPosProtFault_flg_ovrdval"
  Constant: VSRV_TMOverTempIn_flg_ovrdval/1 -> inputs_bus/94  "VSRV_TMOverTempIn_flg_ovrdval"
  Constant: VSRV_TMDeratingIn_flg_ovrdval/1 -> inputs_bus/93  "VSRV_TMDeratingIn_flg_ovrdval"
  Constant: VSRV_BrkLightSWPUnlockActiveValidIn_flg_ovrdval/1 -> inputs_bus/92  "VSRV_BrkLightSWPUnlockActiveValidIn_flg_ovrdval"
  Constant: VSRV_BrkLightSWPUnlockActiveIn_flg_ovrdval/1 -> inputs_bus/91  "VSRV_BrkLightSWPUnlockActiveIn_flg_ovrdval"
  Constant: VSRV_WheelRoughRoadValidIn_flg_ovrdval/1 -> inputs_bus/83  "VSRV_WheelRoughRoadValidIn_flg_ovrdval"
  Constant: VSRV_WheelRoughRoadIn_mps2_ovrdval/1 -> inputs_bus/82  "VSRV_WheelRoughRoadIn_mps2_ovrdval"
  Constant: VSRV_VehSpdRawValidIn_flg_ovrdval/1 -> inputs_bus/81  "VSRV_VehSpdRawValidIn_flg_ovrdval"
  Constant: VSRV_VehSpdRawIn_kph_ovrdval/1 -> inputs_bus/80  "VSRV_VehSpdRawIn_kph_ovrdval"
  Constant: VSRV_TMTqAvailMinValidIn_flg_ovrdval/1 -> inputs_bus/79  "VSRV_TMTqAvailMinValidIn_flg_ovrdval"
  Constant: VSRV_TMTqAvailMinIn_Nm_ovrdval/1 -> inputs_bus/78  "VSRV_TMTqAvailMinIn_Nm_ovrdval"
  Constant: VSRV_TMTqAvailMaxValidIn_flg_ovrdval/1 -> inputs_bus/77  "VSRV_TMTqAvailMaxValidIn_flg_ovrdval"
  Constant: VSRV_TMTqAvailMaxIn_Nm_ovrdval/1 -> inputs_bus/76  "VSRV_TMTqAvailMaxIn_Nm_ovrdval"
  Constant: VSRV_TMTqActValidIn_flg_ovrdval/1 -> inputs_bus/75  "VSRV_TMTqActValidIn_flg_ovrdval"
  Constant: VSRV_TMTqActIn_Nm_ovrdval/1 -> inputs_bus/74  "VSRV_TMTqActIn_Nm_ovrdval"
  Constant: VSRV_TMSpdValidIn_flg_ovrdval/1 -> inputs_bus/73  "VSRV_TMSpdValidIn_flg_ovrdval"
  Constant: VSRV_TMSpdRawValidIn_flg_ovrdval/1 -> inputs_bus/72  "VSRV_TMSpdRawValidIn_flg_ovrdval"
  Constant: VSRV_TMSpdRawIn_rpm_ovrdval/1 -> inputs_bus/71  "VSRV_TMSpdRawIn_rpm_ovrdval"
  Constant: VSRV_TMSpdIn_rpm_ovrdval/1 -> inputs_bus/70  "VSRV_TMSpdIn_rpm_ovrdval"
  Constant: VSRV_TMModeIn_enum_ovrdval/1 -> inputs_bus/69  "VSRV_TMModeIn_enum_ovrdval"
  Constant: VSRV_TMInvtCurrIn_A_ovrdval/1 -> inputs_bus/68  "VSRV_TMInvtCurrIn_A_ovrdval"
  Constant: VSRV_TMDiagReqIn_flg_ovrdval/1 -> inputs_bus/67  "VSRV_TMDiagReqIn_flg_ovrdval"
  Constant: VSRV_TMACShortCircReadyIn_flg_ovrdval/1 -> inputs_bus/66  "VSRV_TMACShortCircReadyIn_flg_ovrdval"
  Constant: VSRV_TCRollingCountBESPIn_cnt_ovrdval/1 -> inputs_bus/65  "VSRV_TCRollingCountBESPIn_cnt_ovrdval"
  Constant: VSRV_TCHSC2FrP02ProtFault_flg_ovrdval/1 -> inputs_bus/64  "VSRV_TCHSC2FrP02ProtFault_flg_ovrdval"
  Constant: VSRV_TCHSC2FrP02Active_flg_ovrdval/1 -> inputs_bus/63  "VSRV_TCHSC2FrP02Active_flg_ovrdval"
  Constant: VSRV_TCHSC2FrP01ProtFault_flg_ovrdval/1 -> inputs_bus/62  "VSRV_TCHSC2FrP01ProtFault_flg_ovrdval"
  Constant: VSRV_TCHSC2FrP01Active_flg_ovrdval/1 -> inputs_bus/61  "VSRV_TCHSC2FrP01Active_flg_ovrdval"
  Constant: VSRV_ShifterPosIn_enum_ovrdval/1 -> inputs_bus/60  "VSRV_ShifterPosIn_enum_ovrdval"
  Constant: VSRV_ShifterInitIn_flg_ovrdval/1 -> inputs_bus/59  "VSRV_ShifterInitIn_flg_ovrdval"
  Constant: VSRV_ShifterFailIn_flg_ovrdval/1 -> inputs_bus/58  "VSRV_ShifterFailIn_flg_ovrdval"
  Constant: VSRV_SecurityChksumBESPIn_cnt_ovrdval/1 -> inputs_bus/57  "VSRV_SecurityChksumBESPIn_cnt_ovrdval"
  Constant: VSRV_SCUHSCFrP00ProtFault_flg_ovrdval/1 -> inputs_bus/56  "VSRV_SCUHSCFrP00ProtFault_flg_ovrdval"
  Constant: VSRV_SCUHSCFrP00Active_flg_ovrdval/1 -> inputs_bus/55  "VSRV_SCUHSCFrP00Active_flg_ovrdval"
  Constant: VSRV_LamdLoopActiveIn_flg_ovrdval/1 -> inputs_bus/54  "VSRV_LamdLoopActiveIn_flg_ovrdval"
  Constant: VSRV_KeySwitchStateIGNIn_flg_ovrdval/1 -> inputs_bus/53  "VSRV_KeySwitchStateIGNIn_flg_ovrdval"
  Constant: VSRV_ISGTqAvailMinValidIn_flg_ovrdval/1 -> inputs_bus/52  "VSRV_ISGTqAvailMinValidIn_flg_ovrdval"
  Constant: VSRV_ISGTqAvailMinIn_Nm_ovrdval/1 -> inputs_bus/51  "VSRV_ISGTqAvailMinIn_Nm_ovrdval"
  Constant: VSRV_ISGTqAvailMaxValidIn_flg_ovrdval/1 -> inputs_bus/50  "VSRV_ISGTqAvailMaxValidIn_flg_ovrdval"
  Constant: VSRV_ISGTqAvailMaxIn_Nm_ovrdval/1 -> inputs_bus/49  "VSRV_ISGTqAvailMaxIn_Nm_ovrdval"
  Constant: VSRV_ISGTqActIn_Nm_ovrdval/1 -> inputs_bus/48  "VSRV_ISGTqActIn_Nm_ovrdval"
  Constant: VSRV_ISGSurgeDampActiveIn_flg_ovrdval/1 -> inputs_bus/47  "VSRV_ISGSurgeDampActiveIn_flg_ovrdval"
  Constant: VSRV_ISGSpdIn_rpm_ovrdval/1 -> inputs_bus/46  "VSRV_ISGSpdIn_rpm_ovrdval"
  Constant: VSRV_ISGModeIn_enum_ovrdval/1 -> inputs_bus/45  "VSRV_ISGModeIn_enum_ovrdval"
  Constant: VSRV_ISGDiagReqIn_flg_ovrdval/1 -> inputs_bus/44  "VSRV_ISGDiagReqIn_flg_ovrdval"
  Constant: VSRV_ISGACShortCircReadyIn_flg_ovrdval/1 -> inputs_bus/43  "VSRV_ISGACShortCircReadyIn_flg_ovrdval"
  Constant: VSRV_ISCHSC2FrP04ProtFault_flg_ovrdval/1 -> inputs_bus/42  "VSRV_ISCHSC2FrP04ProtFault_flg_ovrdval"
  Constant: VSRV_ISCHSC2FrP04Active_flg_ovrdval/1 -> inputs_bus/41  "VSRV_ISCHSC2FrP04Active_flg_ovrdval"
  Constant: VSRV_ISCHSC2FrP03ProtFault_flg_ovrdval/1 -> inputs_bus/40  "VSRV_ISCHSC2FrP03ProtFault_flg_ovrdval"
  Constant: VSRV_ISCHSC2FrP03Active_flg_ovrdval/1 -> inputs_bus/39  "VSRV_ISCHSC2FrP03Active_flg_ovrdval"
  Constant: VSRV_GearShiftInhUpValidIn_flg_ovrdval/1 -> inputs_bus/38  "VSRV_GearShiftInhUpValidIn_flg_ovrdval"
  Constant: VSRV_GearShiftInhUpIn_flg_ovrdval/1 -> inputs_bus/37  "VSRV_GearShiftInhUpIn_flg_ovrdval"
  Constant: VSRV_GearShiftInhDownValidIn_flg_ovrdval/1 -> inputs_bus/36  "VSRV_GearShiftInhDownValidIn_flg_ovrdval"
  Constant: VSRV_GearShiftInhDownIn_flg_ovrdval/1 -> inputs_bus/35  "VSRV_GearShiftInhDownIn_flg_ovrdval"
  Constant: VSRV_FuelCutActiveIn_flg_ovrdval/1 -> inputs_bus/34  "VSRV_FuelCutActiveIn_flg_ovrdval"
  Constant: VSRV_ESPTqRedSlowReqIn_Nm_ovrdval/1 -> inputs_bus/33  "VSRV_ESPTqRedSlowReqIn_Nm_ovrdval"
  Constant: VSRV_ESPTqRedFastReqIn_Nm_ovrdval/1 -> inputs_bus/32  "VSRV_ESPTqRedFastReqIn_Nm_ovrdval"
  Constant: VSRV_ESPTqRedControlActiveIn_flg_ovrdval/1 -> inputs_bus/31  "VSRV_ESPTqRedControlActiveIn_flg_ovrdval"
  Constant: VSRV_ESPTqIncSlowReqIn_Nm_ovrdval/1 -> inputs_bus/30  "VSRV_ESPTqIncSlowReqIn_Nm_ovrdval"
  Constant: VSRV_ESPTqIncControlActiveIn_flg_ovrdval/1 -> inputs_bus/29  "VSRV_ESPTqIncControlActiveIn_flg_ovrdval"
  Constant: VSRV_EngTqStandardValidIn_flg_ovrdval/1 -> inputs_bus/28  "VSRV_EngTqStandardValidIn_flg_ovrdval"
  Constant: VSRV_EngTqStandardIn_Nm_ovrdval/1 -> inputs_bus/27  "VSRV_EngTqStandardIn_Nm_ovrdval"
  Constant: VSRV_EngTqModelStatusIn_enum_ovrdval/1 -> inputs_bus/26  "VSRV_EngTqModelStatusIn_enum_ovrdval"
  Constant: VSRV_EngTqMinIn_Nm_ovrdval/1 -> inputs_bus/25  "VSRV_EngTqMinIn_Nm_ovrdval"
  Constant: VSRV_EngTqMaxIn_Nm_ovrdval/1 -> inputs_bus/24  "VSRV_EngTqMaxIn_Nm_ovrdval"
  Constant: VSRV_EngTqIndActValidIn_flg_ovrdval/1 -> inputs_bus/23  "VSRV_EngTqIndActValidIn_flg_ovrdval"
  Constant: VSRV_EngTqIndActIn_Nm_ovrdval/1 -> inputs_bus/22  "VSRV_EngTqIndActIn_Nm_ovrdval"
  Constant: VSRV_EngTqFrictionIn_Nm_ovrdval/1 -> inputs_bus/21  "VSRV_EngTqFrictionIn_Nm_ovrdval"
  Constant: VSRV_EngTqAllowedMinMonIn_Nm_ovrdval/1 -> inputs_bus/20  "VSRV_EngTqAllowedMinMonIn_Nm_ovrdval"
  Constant: VSRV_EngStoppedIn_flg_ovrdval/1 -> inputs_bus/19  "VSRV_EngStoppedIn_flg_ovrdval"
  Constant: VSRV_EngStartCompleteIn_flg_ovrdval/1 -> inputs_bus/18  "VSRV_EngStartCompleteIn_flg_ovrdval"
  Constant: VSRV_EngSpdValidIn_flg_ovrdval/1 -> inputs_bus/17  "VSRV_EngSpdValidIn_flg_ovrdval"
  Constant: VSRV_EngSpdMonIn_rpm_ovrdval/1 -> inputs_bus/16  "VSRV_EngSpdMonIn_rpm_ovrdval"
  Constant: VSRV_EngSpdIn_rpm_ovrdval/1 -> inputs_bus/15  "VSRV_EngSpdIn_rpm_ovrdval"
  Constant: VSRV_EngIdleIn_flg_ovrdval/1 -> inputs_bus/14  "VSRV_EngIdleIn_flg_ovrdval"
  Constant: VSRV_EMSHSCFrP07ProtFault_flg_ovrdval/1 -> inputs_bus/13  "VSRV_EMSHSCFrP07ProtFault_flg_ovrdval"
  Constant: VSRV_EMSHSCFrP07Active_flg_ovrdval/1 -> inputs_bus/12  "VSRV_EMSHSCFrP07Active_flg_ovrdval"
  Constant: VSRV_EMSHSCFrP00Active_flg_ovrdval/1 -> inputs_bus/11  "VSRV_EMSHSCFrP00Active_flg_ovrdval"
  Constant: VSRV_DSCHSCFrP02ProtFault_flg_ovrdval/1 -> inputs_bus/10  "VSRV_DSCHSCFrP02ProtFault_flg_ovrdval"
  Constant: VSRV_DSCHSCFrP02Active_flg_ovrdval/1 -> inputs_bus/9  "VSRV_DSCHSCFrP02Active_flg_ovrdval"
  Constant: VSRV_DSCHSCFrP00Active_flg_ovrdval/1 -> inputs_bus/8  "VSRV_DSCHSCFrP00Active_flg_ovrdval"
  Constant: VSRV_CruiseTqReqIn_Nm_ovrdval/1 -> inputs_bus/7  "VSRV_CruiseTqReqIn_Nm_ovrdval"
  Constant: VSRV_BrkLightSwitchActiveValidIn_flg_ovrdval/1 -> inputs_bus/6  "VSRV_BrkLightSwitchActiveValidIn_flg_ovrdval"
  Constant: VSRV_BrkLightSwitchActiveIn_flg_ovrdval/1 -> inputs_bus/5  "VSRV_BrkLightSwitchActiveIn_flg_ovrdval"
  Constant: VSRV_BrakePressureValidIn_flg_ovrdval/1 -> inputs_bus/4  "VSRV_BrakePressureValidIn_flg_ovrdval"
  Constant: VSRV_BrakePressureIn_bar_ovrdval/1 -> inputs_bus/3  "VSRV_BrakePressureIn_bar_ovrdval"
  Constant: VSRV_ABSDSCHSCFrP03Active_flg_ovrdval/1 -> inputs_bus/2  "VSRV_ABSDSCHSCFrP03Active_flg_ovrdval"
  Constant: VSRV_ABSDSCHSCFrP00Active_flg_ovrdval/1 -> inputs_bus/1  "VSRV_ABSDSCHSCFrP00Active_flg_ovrdval"
  inputs_bus/1 -> output_bus/1  "output_bus_ovrdval"
  Constant: VSRV_CruiseControlActiveIn_flg_ovrdval/1 -> inputs_bus/84  "VSRV_CruiseControlActiveIn_flg_ovrdval"
  Constant: VSRV_AccelPedalPosnMonIn_pct_ovrdval/1 -> inputs_bus/85  "VSRV_AccelPedalPosnIn_pct_ovrdval"
  Constant: VSRV_CatLightOffReqIn_flg_ovrdval/1 -> inputs_bus/86  "VSRV_CatLightOffReqIn_flg_ovrdval"
  Constant: VSRV_ISGInvtCurrIn_A_ovrdval/1 -> inputs_bus/87  "VSRV_ISGInvtCurrIn_A_ovrdval"
  Constant:VSRV_EMSFltLevelIn_enum_ovrdval/1 -> inputs_bus/88  "VSRV_EMSFltLevelIn_enum_ovrdval"
  Constant: VSRV_IgnitionOnIn_flg_ovrdval/1 -> inputs_bus/89  "VSRV_IgnitionOnIn_flg_ovrdval"
  Constant: VSRV_CrankActiveIn_flg_ovrdval/1 -> inputs_bus/90  "VSRV_CrankActiveIn_flg_ovrdval"

== system inp/INP/INP_10MS/HW_HCU_10ms ==
  BHAL_IN_10ms : Inport
  BSRV_In_ovrdflgs : Inport  Port=2
  BSRV_In_ovrdvals : Inport  Port=3
  Bus Creator : BusCreator  Inputs=2
  Bus Selector10 : BusSelector  OutputSignals=VSRV_CrankActiveIn_flg_ovrdval
  Bus Selector14 : BusSelector  OutputSignals=VSRV_CrankActiveIn_flg_ovrdflg
  Bus Selector15 : BusSelector  OutputSignals=VSRV_IgnitionOnIn_flg_ovrdval
  Bus Selector16 : BusSelector  OutputSignals=VHAL_IgnitionOnIn_flg
  Bus Selector17 : BusSelector  OutputSignals=VSRV_IgnitionOnIn_flg_ovrdflg
  Bus Selector6 : BusSelector  OutputSignals=VHAL_CrankActiveIn_flg
  Subsys VINP_CrankActive_flg : inp_lib/override  SystemSampleTime=-1  cal_ovrdflg=KINP_CrankActive_flg_ovrdflg  cal_ovrdval=KINP_CrankActive_flg_ovrdval
  Subsys VINP_IgnitionOn_flg : inp_lib/override  SystemSampleTime=-1  cal_ovrdflg=KINP_IgnitionOn_flg_ovrdflg  cal_ovrdval=KINP_IgnitionOn_flg_ovrdval
  BINP_HW_HCU_10ms : Outport
  wires:
  Bus Creator/1 -> BINP_HW_HCU_10ms/1  "BINP_HW_HCU_10ms"
  BSRV_In_ovrdflgs/1 -> [BSRV_In_ovrdflgs]
  BSRV_In_ovrdvals/1 -> [BSRV_In_ovrdvals]
  [BSRV_In_ovrdvals] -> Bus Selector15/1
  [BSRV_In_ovrdflgs] -> Bus Selector17/1
  [BSRV_In_ovrdvals] -> Bus Selector10/1
  [BSRV_In_ovrdflgs] -> Bus Selector14/1
  BHAL_IN_10ms/1 -> Bus Selector6/1, Bus Selector16/1
  Bus Selector6/1 -> Subsys VINP_CrankActive_flg/1  "<VHAL_CrankActiveIn_flg>"
  Bus Selector14/1 -> Subsys VINP_CrankActive_flg/2  "<VSRV_CrankActiveIn_flg_ovrdflg>"
  Bus Selector10/1 -> Subsys VINP_CrankActive_flg/3  "<VSRV_CrankActiveIn_flg_ovrdval>"
  Subsys VINP_CrankActive_flg/1 -> Bus Creator/1  "VINP_CrankActive_flg"
  Bus Selector16/1 -> Subsys VINP_IgnitionOn_flg/1  "<VHAL_IgnitionOnIn_flg>"
  Bus Selector17/1 -> Subsys VINP_IgnitionOn_flg/2  "<VSRV_IgnitionOnIn_flg_ovrdflg>"
  Bus Selector15/1 -> Subsys VINP_IgnitionOn_flg/3  "<VSRV_IgnitionOnIn_flg_ovrdval>"
  Subsys VINP_IgnitionOn_flg/1 -> Bus Creator/2  "VINP_IgnitionOn_flg"

== system inp/INP/INP_10MS/Message (10ms) ABS_DSC_HSC_FrP00 ==
  BHAL_IN_10ms : Inport
  BSRV_In_ovrdflgs : Inport  Port=2
  BSRV_In_ovrdvals : Inport  Port=3
  VINP_DSCMsgAlive_flg : Inport  Port=4
  Abs : Abs  OutDataType=fixdt(1, 16)  OutScaling=2^0
  Bus Selector1 : BusSelector  OutputSignals=VSRV_ABSDSCHSCFrP00Active_flg_ovrdval
  Bus Selector10 : BusSelector  OutputSignals=VSRV_VehSpdRawIn_kph_ovrdval
  Bus Selector11 : BusSelector  OutputSignals=VSRV_WheelRoughRoadIn_mps2_ovrdflg
  Bus Selector2 : BusSelector  OutputSignals=VSRV_ABSDSCHSCFrP00Active_flg_ovrdflg
  Bus Selector4 : BusSelector  OutputSignals=VSRV_WheelRoughRoadIn_mps2_ovrdval
  Bus Selector7 : BusSelector  OutputSignals=VHAL_VehSpdRawIn_kph,VHAL_VehSpdRawValidIn_flg
  Bus Selector8 : BusSelector  OutputSignals=VHAL_WheelRoughRoadIn_mps2,VHAL_WheelRoughRoadValidIn_flg
  Bus Selector9 : BusSelector  OutputSignals=VSRV_VehSpdRawIn_kph_ovrdflg
  Subsys VINP_ABSDSCHSCFrP00Active_flg : inp_lib/override  SystemSampleTime=-1  cal_ovrdflg=KINP_ABSDSCHSCFrP00Active_ovrdflg  cal_ovrdval=KINP_ABSDSCHSCFrP00Active_flg_ovrdval
  Subsys VINP_VehSpdRaw_kph : inp_lib/valid_msgactv_sat_ovrd  SystemSampleTime=-1  cal_ovrdflg=KINP_VehSpdRaw_kph_ovrdflg  cal_ovrdval=KINP_VehSpdRaw_kph_ovrdval  lim=KINP_ValidCheck_VehSpdRaw_lim  inc=KINP_ValidCheck_VehSpdRaw_inc  dec=KINP_ValidCheck_VehSpdRaw_dec  default=KINP_VehSpdRawDefault_kph  hi=KINP_VehSpdRawABS_kph_Max  lo=KINP_VehSpdRawABS_kph_Min
  Subsys VINP_WheelRoughRoad_mps2 : inp_lib/valid_msgactv_sat_ovrd  SystemSampleTime=-1  cal_ovrdflg=KINP_WheelRoughRoad_mps2_ovrdflg  cal_ovrdval=KINP_WheelRoughRoad_mps2_ovrdval  lim=KINP_ValidCheck_WheelRoughRoad_lim  inc=KINP_ValidCheck_WheelRoughRoad_inc  dec=KINP_ValidCheck_WheelRoughRoad_dec  default=KINP_WheelRoughRoadDefault_mps2  hi=KINP_WheelRoughRoad_mps2_Max  lo=KINP_WheelRoughRoad_mps2_Min
  inputs_bus1 : BusCreator  Inputs=5
  BINP_ABS_DSC_HSC_FrP00 : Outport  OutDataType=sfix(16)  OutScaling=2^0
  wires:
  [BSRV_In_ovrdflgs] -> Bus Selector11/1
  [BSRV_In_ovrdvals] -> Bus Selector4/1
  inputs_bus1/1 -> BINP_ABS_DSC_HSC_FrP00/1  "BINP_ABS_DSC_HSC_FrP00"
  BSRV_In_ovrdvals/1 -> [BSRV_In_ovrdvals]
  BSRV_In_ovrdflgs/1 -> [BSRV_In_ovrdflgs]
  VINP_DSCMsgAlive_flg/1 -> [VINP_DSCMsgAlive_flg]
  BHAL_IN_10ms/1 -> Bus Selector8/1, Bus Selector7/1
  [BSRV_In_ovrdflgs] -> Bus Selector9/1
  [BSRV_In_ovrdvals] -> Bus Selector10/1
  Bus Selector7/1 -> Abs/1  "<VHAL_VehSpdRawIn_kph>"
  [VINP_DSCMsgAlive_flg] -> [MsgAlive_flgs], Subsys VINP_ABSDSCHSCFrP00Active_flg/1
  [BSRV_In_ovrdflgs] -> Bus Selector2/1
  [BSRV_In_ovrdvals] -> Bus Selector1/1
  Bus Selector2/1 -> Subsys VINP_ABSDSCHSCFrP00Active_flg/2  "<VSRV_ABSDSCHSCFrP00Active_flg_ovrdflg>"
  Bus Selector1/1 -> Subsys VINP_ABSDSCHSCFrP00Active_flg/3  "<VSRV_ABSDSCHSCFrP00Active_flg_ovrdval>"
  Subsys VINP_ABSDSCHSCFrP00Active_flg/1 -> inputs_bus1/5  "VINP_ABSDSCHSCFrP00Active_flg"
  Bus Selector8/1 -> Subsys VINP_WheelRoughRoad_mps2/1  "<VHAL_WheelRoughRoadIn_mps2>"
  Bus Selector8/2 -> Subsys VINP_WheelRoughRoad_mps2/2  "<VHAL_WheelRoughRoadValidIn_flg>"
  Bus Selector11/1 -> Subsys VINP_WheelRoughRoad_mps2/3  "<VSRV_WheelRoughRoadIn_mps2_ovrdflg>"
  Bus Selector4/1 -> Subsys VINP_WheelRoughRoad_mps2/4  "<VSRV_WheelRoughRoadIn_mps2_ovrdval>"
  [MsgAlive_flgs] -> Subsys VINP_WheelRoughRoad_mps2/5
  Subsys VINP_WheelRoughRoad_mps2/1 -> inputs_bus1/3  "VINP_WheelRoughRoad_mps2"
  Subsys VINP_WheelRoughRoad_mps2/2 -> inputs_bus1/4  "VINP_WheelRoughRoadValid_flg"
  Abs/1 -> Subsys VINP_VehSpdRaw_kph/1
  Bus Selector7/2 -> Subsys VINP_VehSpdRaw_kph/2  "<VHAL_VehSpdRawValidIn_flg>"
  Bus Selector9/1 -> Subsys VINP_VehSpdRaw_kph/3  "<VSRV_VehSpdRawIn_kph_ovrdflg>"
  Bus Selector10/1 -> Subsys VINP_VehSpdRaw_kph/4  "<VSRV_VehSpdRawIn_kph_ovrdval>"
  [MsgAlive_flgs] -> Subsys VINP_VehSpdRaw_kph/5
  Subsys VINP_VehSpdRaw_kph/1 -> inputs_bus1/1  "VINP_VehSpdRawABS_kph"
  Subsys VINP_VehSpdRaw_kph/2 -> inputs_bus1/2  "VINP_VehSpdRawValid_flg"
